simulink model "resonant_pulse_commutation"  (R2022b)
settings: Solver=VariableStepAuto  StartTime=0.0  StopTime=1  RelTol=1e-3
libraries: spsSeriesRLCBranchLib x2, spsThyristorLib x2, spsCurrentMeasurementLib x1, spsDCVoltageSourceLib x1, spsDiodeLib x1, spsVoltageMeasurementLib x1, sps_lib x1
settings Model: Creator=Shantanu  LastModifiedBy=Shantanu

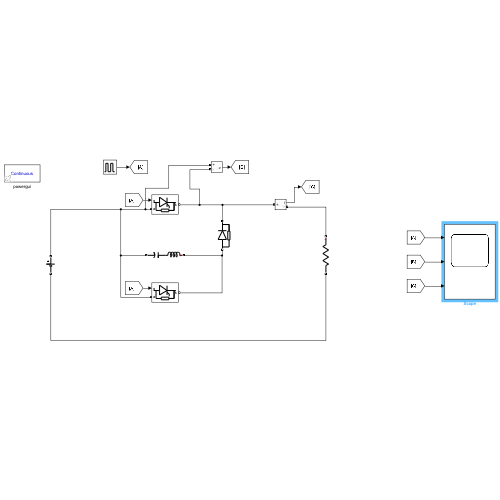
[thumbnail: Simulink's stored preview of the top-level diagram]
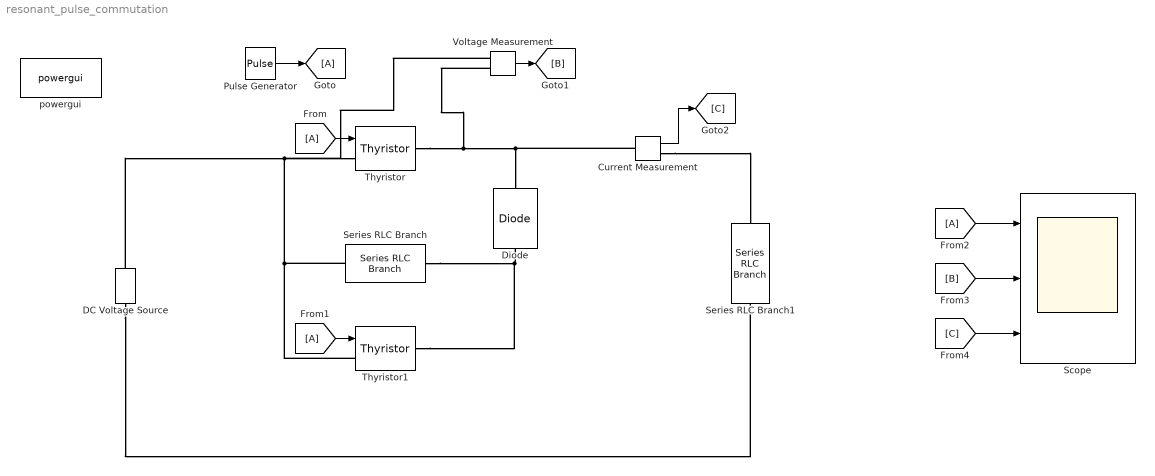
== system resonant_pulse_commutation ==
  Current Measurement : spsCurrentMeasurementLib/Current Measurement  PhasorSimulation=off  OutputType=Complex  PSBequivalent=0
  DC Voltage Source : spsDCVoltageSourceLib/DC Voltage Source  Amplitude=230  Measurements=None
  Diode : spsDiodeLib/Diode  Ron=0.001  Lon=0  Vf=0.8  IC=0  UseSnubber=0  Rs=500  Cs=250e-9  Measurements=off
  From : From
  From1 : From
  From2 : From
  Goto : Goto
  Pulse Generator : DiscretePulseGenerator  PulseType=Time based  Amplitude=100  Period=62.8e-6  PulseWidth=5
  Scope : Scope  NumInputPorts=3
  Series RLC Branch : spsSeriesRLCBranchLib/Series RLC Branch  LConnTagsString=__new0  RConnTagsString=__new0  BranchType=LC  Resistance=1  Inductance=5e-6  SetiL0=off  InitialCurrent=0  Capacitance=20e-6  Setx0=on  InitialVoltage=230  Measurements=None
  Series RLC Branch1 : spsSeriesRLCBranchLib/Series RLC Branch  LConnTagsString=__new0  RConnTagsString=__new0  BranchType=R  Resistance=1  Inductance=1e-3  SetiL0=off  InitialCurrent=0  Capacitance=1e-6  Setx0=off  InitialVoltage=0  Measurements=None
  Thyristor : spsThyristorLib/Thyristor  Ron=0.001  Lon=0  Vf=0.8  IC=0  Rs=500  Cs=250e-9  Measurements=off
  Thyristor1 : spsThyristorLib/Thyristor  Ron=0.001  Lon=0  Vf=0.8  IC=0  Rs=500  Cs=250e-9  Measurements=off
  Voltage Measurement : spsVoltageMeasurementLib/Voltage Measurement  PhasorSimulation=off  OutputType=Complex  PSBequivalent=0
  powergui : sps_lib/powergui  Priority=1  SimulationMode=Continuous  SampleTime=50e-6  frequency=60  Iterations=50  frequencyindice=0  Pbase=100e6  ErrMax=1e-4  UnitsV=kV  UnitsW=MW  buscounter=0  FunctionMessages=off  echomessages=off  EnableUseOfTLC=off  CurrentSourceSwitches=off  DisableSnubberDevices=off  DisableRonSwitches=off  DisableVfSwitches=off  DisplayEquations=off  AutomaticDiscreteSolvers=off  SolverType=Tustin/Backward Euler (TBE)  Interpol=off  ExternalGateDelay=off  methode=off  Ts=100  x0status=blocks  SPID=on  SwTol=0  HookPort=off  NonlinearTolerance=1e-4  nMaxIteration=100  ContinueOnMaxIteration=off  RestoreLinks=warning  ResistiveCurrentMeasurement=off  Frange=[0:2:500]  Ylog=off  Xlog=on  ShowGrid=off  save=off  variable=ZData  structure=0  ZoomFFT=off  StartTime=0.0  cycles=1  DisplayStyle=1  fundamental=60  FreqAxis=off  MaxFrequency=1000  frequencyindicesteady=1  RmsSteady=1  display=off
  wires:
  Pulse Generator/1 -> Goto/1
  From/1 -> Thyristor/1
  From1/1 -> Thyristor1/1
  Voltage Measurement/1 -> [B]
  From2/1 -> Scope/1
  [B] -> Scope/2
  Current Measurement/1 -> [C]
  [C] -> Scope/3
  connections:
  Thyristor/RConn1 -- Voltage Measurement/LConn2 -- Current Measurement/LConn1 -- Diode/RConn1
  Series RLC Branch/LConn1 -- Thyristor1/RConn1 -- Diode/LConn1
  Thyristor1/LConn1 -- DC Voltage Source/RConn1 -- Voltage Measurement/LConn1 -- Thyristor/LConn1 -- Series RLC Branch/RConn1
  DC Voltage Source/LConn1 -- Series RLC Branch1/RConn1
  Current Measurement/RConn1 -- Series RLC Branch1/LConn1
